simulink model "deadbeat_smm_with_lqr"  (R2015a)
settings: Solver=FixedStepDiscrete  SolverMode=SingleTasking  StartTime=0.0  StopTime=inf  FixedStep=sample_time  RelTol=1e-3
undefined symbols (not defined in the file or in its folder): A_kalman_fourbar_gear, A_kalman_transverse, A_kalman_vertical, A_lpf_accelerometer, A_lpf_fourbar_angles, A_lpf_imu, A_lpf_lateral_angle, B1_lpf_accelerometer, B1_lpf_fourbar_angles, B1_lpf_imu, B1_lpf_lateral_angle, B2_lpf_accelerometer, B2_lpf_fourbar_angles, B2_lpf_imu, B2_lpf_lateral_angle, B_dx_versus_x0, B_kalman_fourbar_gear, B_kalman_transverse, B_kalman_vertical, backwards_K_sag_of_t, backwards_P_sag_of_t, C_kalman_fourbar_gear, C_kalman_transverse, C_kalman_vertical, com_leg_motor, com_torso, contact_threshold, control_start_time, d_ankle_to_foot, d_vertical_com, desired_com_forward_velocity, desired_com_lateral_velocity, desired_initial_leg_roll_left, desired_initial_leg_roll_right, desired_stance_beta2, desired_standing_torso_pitch, desired_standing_torso_roll, desired_standing_z, desired_torso_pitch, desired_torso_roll, Discrete, enable_bouncing, fcut_contact, fdesignblkfcn, forward_dx_of_dxstar, forward_x_of_dxstar, g, gcbh, HIP_MTR_MAX_CONT_TORQUE, HIP_MTR_MAX_TORQUE, i_leg_motor, i_robot, i_torso, initial_dx_estimate, initial_dy_estimate, initial_dz_estimate, initial_leg_selection, initial_z_estimate, k_lateral_accel_for_torso_roll, k_lateral_swing_on_boom ... (+77)
libraries: simulink x21, ctrlSharedLib x7, dsparch4 x3
(part 1 of 5)
settings Model: CovSFcnEnable=off  Creator=wmartin  LastModifiedBy=wmartin
settings SolverCC: EnableConcurrentExecution=on
settings DataIOCC: LimitDataPoints=off  MaxDataPoints=1000000000  SaveFormat=StructureWithTime  SignalLogging=off  DSMLogging=off  VisualizeSimOutput=off
settings OptimizationCC: BlockReduction=off  OptimizeBlockIOStorage=off  BufferReuse=off  GlobalBufferReuse=off  ExpressionFolding=off  ExpressionDepthLimit=2147483647  LocalBlockOutputs=off  SimCompilerOptimization=on
settings DebuggingCC: UnderspecifiedInitializationDetection=Classic  MergeDetectMultiDrivingBlocksExec=none  SolverPrmCheckMsg=warning  StateNameClashWarn=warning
settings HardwareCC: ProdIntDivRoundTo=Zero  ProdEndianess=LittleEndian  ProdLongLongMode=on  ProdHWDeviceType=Generic->32-bit x86 compatible
settings ModelReferenceCC: UpdateModelReferenceTargets=IfOutOfDate  ModelReferenceNumInstancesAllowed=Single  ModelReferenceMinAlgLoopOccurrences=on
settings RTWCC: SystemTargetFile=slrt.tlc  TemplateMakefile=slrt_default_tmf  Description=Simulink Real-Time  RTWVerbose=off  RTWCompilerOptimization=on
settings CodeAppCC: MaxIdLength=256
settings SimulinkRealTimeCC: GeneratePreprocessorConditionals=Disable all  RL32LogBufSizeModifier=1e8

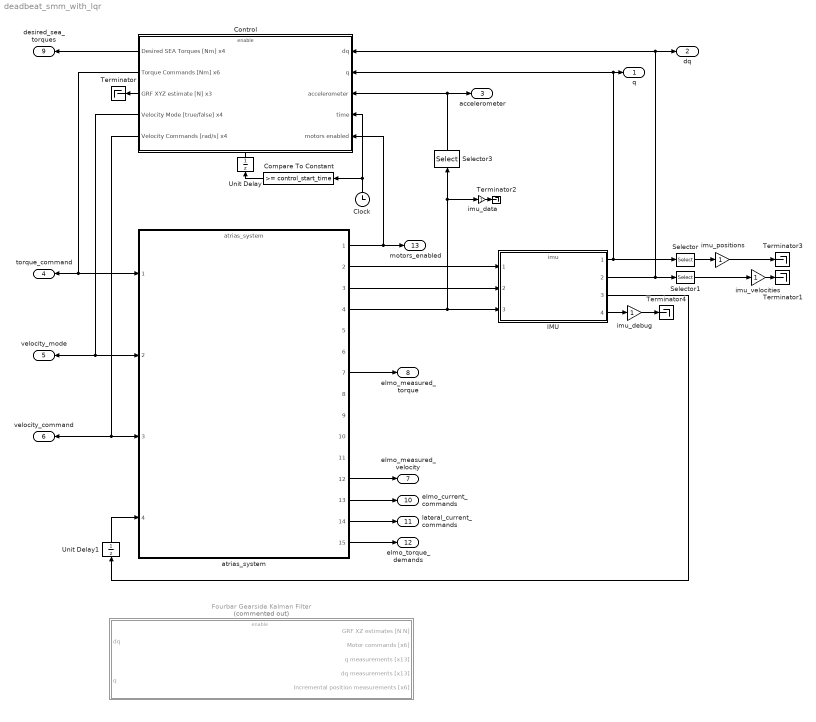
== system deadbeat_smm_with_lqr ==
  Clock : Clock
  Compare To Constant : simulink/Logic and Bit Operations/Compare To Constant  relop=>=  const=control_start_time  OutDataTypeStr=boolean
  Control : Subsystem
  Fourbar Gearside Kalman Filter : Subsystem  Commented=on
  IMU : ModelReference  ModelNameDialog=imu  SimulationMode=Normal  ModelReferenceVersion=1.2455  CopyOfModelName=imu  DefaultDataLogging=on
  Selector : Selector  InputPortWidth=13  Indices=[11 12 13]
  Selector1 : Selector  InputPortWidth=13  Indices=[11 12 13]
  Selector3 : Selector  InputPortWidth=9  Indices=[4 5 6]
  Terminator{,1..4} (5 alike) : Terminator
  Unit Delay : UnitDelay  SampleTime=-1
  Unit Delay1 : UnitDelay  SampleTime=-1
  atrias_system : ModelReference  ModelNameDialog=atrias_system  SimulationMode=Normal  ModelReferenceVersion=1.2965  CopyOfModelName=atrias_system  DefaultDataLogging=on
  imu_data : Gain
  imu_debug : Gain
  imu_positions : Gain
  imu_velocities : Gain
  q : Outport  SampleTime=sample_time
  dq : Outport  Port=2  SampleTime=sample_time
  accelerometer : Outport  Port=3  SampleTime=sample_time
  torque_command : Outport  Port=4  SampleTime=sample_time
  velocity_mode : Outport  Port=5  SampleTime=sample_time
  velocity_command : Outport  Port=6  SampleTime=sample_time
  elmo_measured_velocity : Outport  Port=7  SampleTime=sample_time
  elmo_measured_torque : Outport  Port=8  SampleTime=sample_time
  desired_sea_torques : Outport  Port=9  SampleTime=sample_time
  elmo_current_commands : Outport  Port=10  SampleTime=sample_time
  lateral_current_commands : Outport  Port=11  SampleTime=sample_time
  elmo_torque_demands : Outport  Port=12  SampleTime=sample_time
  motors_enabled : Outport  Port=13  SampleTime=sample_time
  wires:
  Compare To Constant/1 -> Unit Delay/1
  imu_data/1 -> Terminator2/1
  imu_velocities/1 -> Terminator1/1
  imu_positions/1 -> Terminator3/1
  imu_debug/1 -> Terminator4/1
  IMU/4 -> imu_debug/1
  Selector/1 -> imu_positions/1
  Selector1/1 -> imu_velocities/1
  atrias_system/2 -> IMU/1
  IMU/1 -> Selector/1, Control/2(q), q/1
  Control/2(Torque Commands [Nm] x6) -> atrias_system/1, torque_command/1
  atrias_system/3 -> IMU/2
  atrias_system/4 -> Selector3/1, imu_data/1, IMU/3
  IMU/3 -> Unit Delay1/1
  Unit Delay/1 -> Control/Enable
  IMU/2 -> Selector1/1, Control/1(dq), dq/1
  Control/5(Velocity Commands [rad/s] x4) -> velocity_command/1, atrias_system/3
  Control/4(Velocity Mode [true/false] x4) -> velocity_mode/1, atrias_system/2
  Selector3/1 -> Control/3(accelerometer), accelerometer/1
  Control/1(Desired SEA Torques [Nm] x4) -> desired_sea_torques/1
  Clock/1 -> Control/4(time), Compare To Constant/1
  Control/3(GRF XYZ estimate [N] x3) -> Terminator/1
  atrias_system/15 -> elmo_torque_demands/1
  atrias_system/14 -> lateral_current_commands/1
  atrias_system/13 -> elmo_current_commands/1
  atrias_system/12 -> elmo_measured_velocity/1
  atrias_system/7 -> elmo_measured_torque/1
  atrias_system/1 -> Control/5(motors enabled), motors_enabled/1
  Unit Delay1/1 -> atrias_system/4

== system deadbeat_smm_with_lqr/Control ==
  dq : Inport
  q : Inport  Port=2
  accelerometer : Inport  Port=3
  time : Inport  Port=4
  motors enabled : Inport  Port=5
  Enable : EnablePort  StatesWhenEnabling=reset  PropagateVarSize=During execution  ShowOutputPort=on
  Actuator Control : ModelReference  ModelNameDialog=actuator_control  SimulationMode=Normal  ModelReferenceVersion=1.1251  CopyOfModelName=actuator_control  DefaultDataLogging=on
  Behavior Control : Subsystem
  Compute Body Frame Accelerations : Subsystem
  Detect Change : simulink/Logic and Bit Operations/Detect Change  vinit=0  InputProcessing=Inherited  OutDataTypeStr=boolean
  Filter Velocities : Subsystem
  Mux : Mux
  Desired SEA Torques [Nm] x4 : Outport  InitialOutput=[0 0 0 0]
  Torque Commands [Nm] x6 : Outport  Port=2  InitialOutput=[0 0 0 0 0 0]
  GRF XYZ estimate [N] x3 : Outport  Port=3  InitialOutput=[0 0 0]
  Velocity Mode [true/false] x4 : Outport  Port=4  InitialOutput=[false false false false]
  Velocity Commands [rad/s] x4 : Outport  Port=5  InitialOutput=[0 0 0 0]
  wires:
  Behavior Control/1(Torque Commands [Nm] x6) -> Actuator Control/2
  Behavior Control/2(Velocity Commands [rad/s] x4) -> Actuator Control/3
  Behavior Control/3(Stance / Swing Control [1/0] x4) -> Actuator Control/4
  time/1 -> Actuator Control/5, Behavior Control/5(time)
  Detect Change/1 -> Mux/1, Mux/2, Mux/3, Mux/4
  motors enabled/1 -> Detect Change/1
  Mux/1 -> Actuator Control/1
  Actuator Control/4 -> Desired SEA Torques [Nm] x4/1
  Enable/1 -> Behavior Control/1(Enabled [true/false])
  Compute Body Frame Accelerations/1(accelerations [m/s^2] x3) -> Behavior Control/2(Body XYZ Acceleration [m/s^2] x3)
  accelerometer/1 -> Compute Body Frame Accelerations/1(accelerometer [g] x3)
  Actuator Control/3 -> Velocity Commands [rad/s] x4/1
  Actuator Control/2 -> Velocity Mode [true/false] x4/1
  dq/1 -> Actuator Control/7, Filter Velocities/1(raw dq)
  Filter Velocities/1(filtered dq) -> Behavior Control/3(dq)
  Behavior Control/4(GRF XYZ estimates [N N N]) -> GRF XYZ estimate [N] x3/1
  Actuator Control/1 -> Torque Commands [Nm] x6/1
  q/1 -> Actuator Control/6, Behavior Control/4(q)

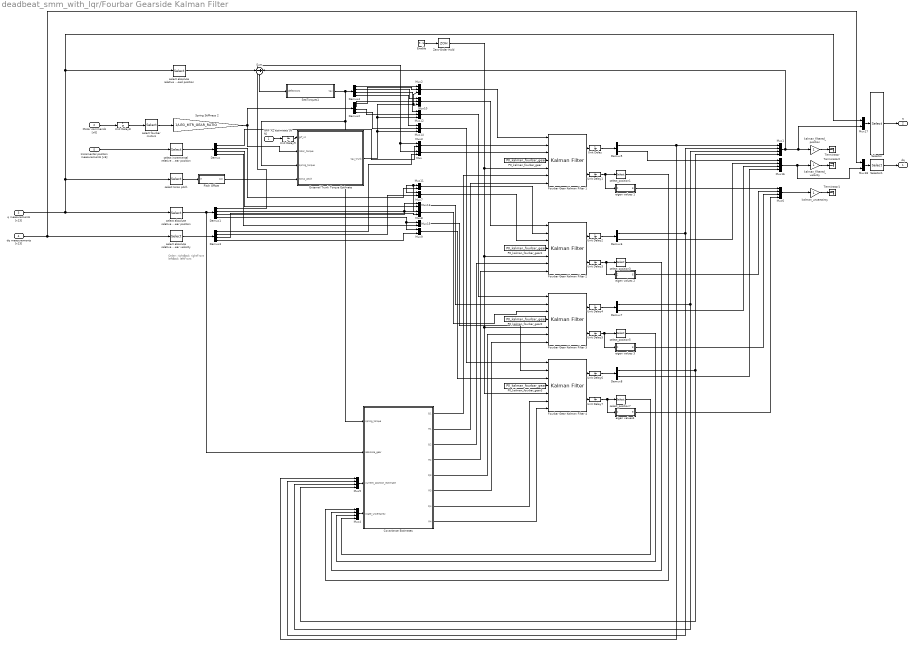
== system deadbeat_smm_with_lqr/Fourbar Gearside Kalman Filter ==
  note: Order:
      | rightBack
      | rightFront
      | leftBack
      | leftFront
  GRF XZ estimates [N N] : Inport  SampleTime=sample_time
  Motor commands [x6] : Inport  Port=2  SampleTime=sample_time
  q measurements [x13] : Inport  Port=3  SampleTime=sample_time
  dq measurements [x13] : Inport  Port=4  SampleTime=sample_time
  Incremental position measurements [x6] : Inport  Port=5  SampleTime=sample_time
  Enable : EnablePort  ShowOutputPort=on
  Covariance Estimates : MATLAB Function  TreatAsAtomicUnit=on
  Demux{,1..4} (5 alike) : Demux
  Demux{5..8} (4 alike) : Demux  Outputs=2
  External Trunk Torque Estimate : MATLAB Function  TreatAsAtomicUnit=on
  Fourbar Gear Kalman Filter {1..4} (4 alike) : ctrlSharedLib/Kalman Filter  TimeDomain=Discrete-Time  UseCurrentEstimator=on  ModelSource=Individual A, B, C, D matrices  ModelSourceVariable=A_kf  A=A_kalman_fourbar_gear  B=B_kalman_fourbar_gear  C=C_kalman_fourbar_gear  D=0  NumberOfStates=2  NumberOfInputs=1  NumberOfOutputs=2  InitialEstimateSource=Input port  X0=initial_dx_estimate  P0=P0_kalman_transverse  UseK=off  UseGH=on  NumberOfProcessNoiseInputs=1  G=G_kalman_fourbar_gear  TimeInvariantG=on  H=0  TimeInvariantH=on  Q=1  TimeInvariantQ=off  R=1  TimeInvariantR=off  N=0  TimeInvariantN=on  AddInputPort=on  AddEnablePort=off  ExternalReset=Either  OutputEstimatedY=off  OutputP=on  Ts=sample_time
  Mux{,3,7..9,11,13,15,17..18} (10 alike) : Mux  Inputs=2
  Mux{1,4..6,16} (5 alike) : Mux
  Mux{2,10,12,14} (4 alike) : Mux  Inputs=3
  P0_kalman_fourbar_gear{,1..3} (4 alike) : Constant  Value=P0_kalman_fourbar_gear
  Pitch Offset : Subsystem
  SeaTorques1 : MATLAB Function  TreatAsAtomicUnit=on
  Selector : Selector  InputPortWidth=17  Indices=[1 14 3 15 5 16 7 17 9 10 11 12 13]
  Selector1 : Selector  InputPortWidth=17  Indices=[1 14 3 15 5 16 7 17 9 10 11 12 13]
  Spring Stiffness 2 : Gain  Gain=1/LEG_MTR_GEAR_RATIO
  Sum : Sum  Inputs=-|+
  Terminator : Terminator
  Terminator1 : Terminator
  Terminator2 : Terminator
  Unit Delay{,1..9} (10 alike) : UnitDelay  SampleTime=-1
  Zero-Order Hold : ZeroOrderHold  SampleTime=sample_time
  eigen values 1 : MATLAB Function  TreatAsAtomicUnit=on
  eigen values 2 : MATLAB Function  TreatAsAtomicUnit=on
  eigen values 3 : MATLAB Function  TreatAsAtomicUnit=on
  "eigen values4 " : MATLAB Function  TreatAsAtomicUnit=on
  kalman_filtered_position : Gain
  kalman_filtered_velocity : Gain
  kalman_uncertainty : Gain
  select absolute relative gear position : Selector  InputPortWidth=13  Indices=[2 4 6 8]
  select absolute relative gear velocity : Selector  InputPortWidth=13  Indices=[2 4 6 8]
  select absolute relative load position : Selector  InputPortWidth=13  Indices=[2 4 6 8]
  select fourbar motors : Selector  InputPortWidth=6  Indices=[1 2 3 4]
  select incremental relative gear position : Selector  InputPortWidth=6  Indices=[1 2 3 4]
  select torso pitch : Selector  InputPortWidth=13  Indices=[13]
  select_position{1,3,5,7} (4 alike) : Selector  NumberOfDimensions=2  InputPortWidth=2  IndexOptions=Index vector (dialog),Index vector (dialog)  Indices=[1],[1]  OutputSizes=1,1
  dq : Outport
  q : Outport  Port=2
  wires:
  select incremental relative gear position/1 -> Demux/1
  q measurements [x13]/1 -> select absolute relative gear position/1, Mux17/1, select absolute relative load position/1, select torso pitch/1
  Incremental position measurements [x6]/1 -> select incremental relative gear position/1
  Motor commands [x6]/1 -> Unit Delay8/1
  select fourbar motors/1 -> Spring Stiffness 2/1
  P0_kalman_fourbar_gear/1 -> Fourbar Gear Kalman Filter 1/4
  Mux/1 -> Fourbar Gear Kalman Filter 1/3
  select absolute relative gear velocity/1 -> Demux3/1
  dq measurements [x13]/1 -> Mux18/1, select absolute relative gear velocity/1
  Demux3/1 -> Mux/2
  GRF XZ estimates [N N]/1 -> Unit Delay9/1
  SeaTorques1/1(tau) -> Demux4/1, External Trunk Torque Estimate/3(spring_torque), Covariance Estimates/1(spring_torque)
  Fourbar Gear Kalman Filter 1/1 -> Unit Delay/1
  Demux5/1 -> Mux1/1, Mux5/1
  Mux1/1 -> Sum/2, Mux17/2, kalman_filtered_position/1
  select absolute relative load position/1 -> Sum/1
  Sum/1 -> SeaTorques1/1(deflections)
  External Trunk Torque Estimate/1(tau_trunk) -> Mux2/3, Mux10/3, Mux12/3, Mux14/3
  Demux4/1 -> Mux2/1
  Demux2/1 -> Mux2/2
  Mux2/1 -> Fourbar Gear Kalman Filter 1/1
  Demux/1 -> Mux3/2
  Demux1/1 -> Mux3/1, Mux/1
  Mux3/1 -> Fourbar Gear Kalman Filter 1/2
  Fourbar Gear Kalman Filter 1/2 -> Unit Delay1/1
  Mux4/1 -> Covariance Estimates/4(state_uncertainty)
  select absolute relative gear position/1 -> Covariance Estimates/2(absolute_gear), Demux1/1
  Mux5/1 -> Covariance Estimates/3(current_position_estimate)
  Covariance Estimates/1(Q1) -> Fourbar Gear Kalman Filter 1/6
  Covariance Estimates/2(R1) -> Fourbar Gear Kalman Filter 1/7
  select torso pitch/1 -> Pitch Offset/1(in)
  select_position1/1 -> Mux4/1
  P0_kalman_fourbar_gear1/1 -> Fourbar Gear Kalman Filter 2/4
  Fourbar Gear Kalman Filter 2/1 -> Unit Delay2/1
  Fourbar Gear Kalman Filter 2/2 -> Unit Delay3/1
  P0_kalman_fourbar_gear2/1 -> Fourbar Gear Kalman Filter 3/4
  Fourbar Gear Kalman Filter 3/1 -> Unit Delay4/1
  Fourbar Gear Kalman Filter 3/2 -> Unit Delay5/1
  P0_kalman_fourbar_gear3/1 -> Fourbar Gear Kalman Filter 4/4
  Fourbar Gear Kalman Filter 4/1 -> Unit Delay6/1
  Fourbar Gear Kalman Filter 4/2 -> Unit Delay7/1
  Covariance Estimates/3(Q2) -> Fourbar Gear Kalman Filter 2/6
  Covariance Estimates/5(Q3) -> Fourbar Gear Kalman Filter 3/6
  Covariance Estimates/7(Q4) -> Fourbar Gear Kalman Filter 4/6
  Covariance Estimates/4(R2) -> Fourbar Gear Kalman Filter 2/7
  Covariance Estimates/6(R3) -> Fourbar Gear Kalman Filter 3/7
  Covariance Estimates/8(R4) -> Fourbar Gear Kalman Filter 4/7
  select_position3/1 -> Mux4/2
  select_position5/1 -> Mux4/3
  select_position7/1 -> Mux4/4
  Demux6/1 -> Mux5/2, Mux1/2
  Demux7/1 -> Mux1/3, Mux5/3
  Demux8/1 -> Mux1/4, Mux5/4
  kalman_filtered_position/1 -> Terminator/1
  Enable/1 -> Zero-Order Hold/1
  Mux7/1 -> Fourbar Gear Kalman Filter 2/3
  Mux8/1 -> Fourbar Gear Kalman Filter 3/3
  Mux9/1 -> Fourbar Gear Kalman Filter 4/3
  Mux10/1 -> Fourbar Gear Kalman Filter 2/1
  Mux11/1 -> Fourbar Gear Kalman Filter 2/2
  Mux13/1 -> Fourbar Gear Kalman Filter 3/2
  Mux12/1 -> Fourbar Gear Kalman Filter 3/1
  Mux15/1 -> Fourbar Gear Kalman Filter 4/2
  Mux14/1 -> Fourbar Gear Kalman Filter 4/1
  Demux3/2 -> Mux7/2
  Demux3/3 -> Mux8/2
  Demux3/4 -> Mux9/2
  Demux1/2 -> Mux7/1, Mux11/1
  Demux1/3 -> Mux13/1, Mux8/1
  Demux1/4 -> Mux9/1, Mux15/1
  Demux/2 -> Mux11/2
  Demux/3 -> Mux13/2
  Demux/4 -> Mux15/2
  Demux4/2 -> Mux10/1
  Demux4/3 -> Mux12/1
  Demux4/4 -> Mux14/1
  Demux2/2 -> Mux10/2
  Demux2/3 -> Mux12/2
  Demux2/4 -> Mux14/2
  kalman_uncertainty/1 -> Terminator1/1
  Mux6/1 -> kalman_uncertainty/1
  kalman_filtered_velocity/1 -> Terminator2/1
  Mux16/1 -> Mux18/2, kalman_filtered_velocity/1
  Demux5/2 -> Mux16/1
  Demux6/2 -> Mux16/2
  Demux7/2 -> Mux16/3
  Demux8/2 -> Mux16/4
  Zero-Order Hold/1 -> Fourbar Gear Kalman Filter 4/5, Fourbar Gear Kalman Filter 3/5, Fourbar Gear Kalman Filter 2/5, Fourbar Gear Kalman Filter 1/5
  Unit Delay1/1 -> eigen values 1/1(Z), select_position1/1
  Unit Delay3/1 -> eigen values 2/1(Z), select_position3/1
  Unit Delay4/1 -> Demux7/1
  Unit Delay7/1 -> "eigen values4 "/1(Z), select_position7/1
  Unit Delay6/1 -> Demux8/1
  Spring Stiffness 2/1 -> Demux2/1, External Trunk Torque Estimate/2(rotor_torque)
  Unit Delay5/1 -> eigen values 3/1(Z), select_position5/1
  eigen values 1/1(E) -> Mux6/1
  eigen values 2/1(E) -> Mux6/2
  eigen values 3/1(E) -> Mux6/3
  "eigen values4 "/1(E) -> Mux6/4
  Unit Delay/1 -> Demux5/1
  Unit Delay2/1 -> Demux6/1
  Mux17/1 -> Selector/1
  Selector/1 -> q/1
  Selector1/1 -> dq/1
  Mux18/1 -> Selector1/1
  Unit Delay8/1 -> select fourbar motors/1
  Unit Delay9/1 -> External Trunk Torque Estimate/1(grf_xz)
  Pitch Offset/1(out) -> External Trunk Torque Estimate/4(torso_pitch)

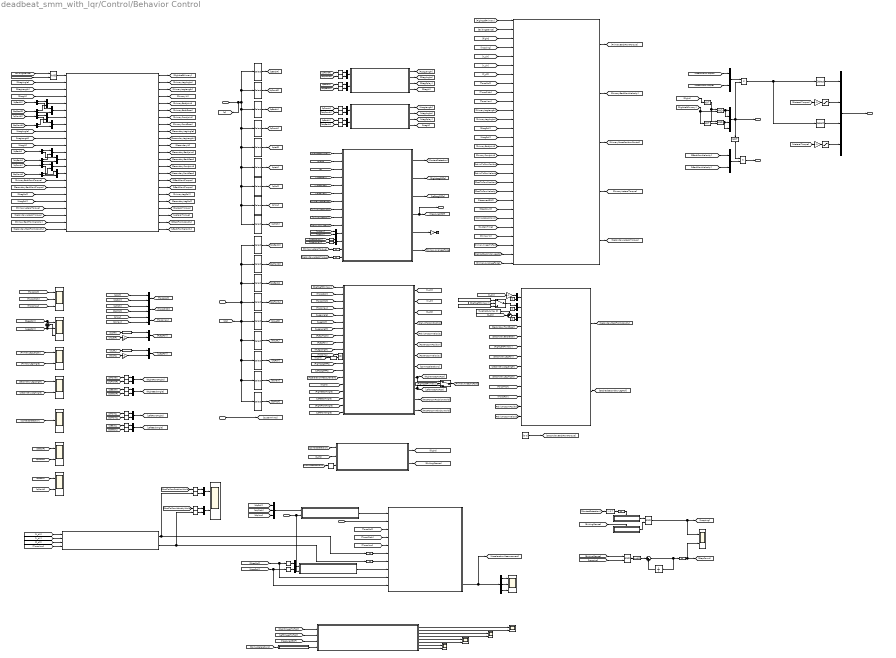
== system deadbeat_smm_with_lqr/Control/Behavior Control ==
  note: Knee Torque Estimation
  note: Acceleration Measurement
  note: Logging
  note: Contact Estimation
  note: Angle Conversions
  note: Motor Order:
      |
      | backR
      | frontR
      | latR
      | backL
      | frontL
      | latL
  note: q Order:
      |
      | backJointR
      | backGearR
      | frontJointR
      | frontGearR
      |
      | backJointL
      | backGearL
      | frontJointL
      | frontGearL
      |
      | latR
      | latL
      |
      | torsoRoll
      | torsoYaw
      | torsoPitch
  note: Inputs
  note: Primary Leg + Lateral Behavior
  note: Secondary Leg Behavior
  note: Torque Commands
  note: Leg/Spring Measurements
  note: Force Estimation
  note: Position & Velocity Estimation
  note: Begin Control
  note: Signal Routing
  Enabled [true/false] : Inport
  Body XYZ Acceleration [m/s^2] x3 : Inport  Port=2
  dq : Inport  Port=3
  q : Inport  Port=4
  time : Inport  Port=5
  At Least One Stance Detected : Subsystem
  Atrias Swing control : Subsystem
  COM Acceleration Measurement : Scope  NumInputPorts=3
      settings: YMin=-10~-12.5~-15  YMax=7.5~7.5~15  SaveName=ScopeData34  SampleInput=on
  COM World Frame X : Scope  NumInputPorts=2
      settings: TimeRange=3.175000000000004  YMin=-0.004~-0.175  YMax=0.02~0.225  SaveName=ScopeData35  SampleInput=on
  Compare To Constant : simulink/Logic and Bit Operations/Compare To Constant  relop=>  const=0.7  OutDataTypeStr=boolean
  Compute COM Translational Acceleration (IMU uses non-rotating measurement frame) : MATLAB Function  TreatAsAtomicUnit=on
  Compute Forces1 : Subsystem
  Compute World Frame COM Coordinates from Yawed Frame : MATLAB Function  TreatAsAtomicUnit=on
  Constant : Constant  Value=[0 0]
  Constant1 : Constant  Value=[lateral_target_position_right, 0]
  Constant2 : Constant  Value=[lateral_target_position_left, 0]
  Constant3 : Constant  Value=[z_retract_swing, 0]
  Constant4 : Constant  Value=0
  Constant5 : Constant  Value=0
  Constant6 : Constant  Value=0
  Contact : Scope
      settings: YMin=0.3  YMax=0.9  SaveName=ScopeData11  SampleInput=on
  Contact State Machine : Subsystem
  Data Type Conversion : DataTypeConversion  OutDataTypeStr=uint32
  Demux : Demux  Outputs=3
  Demux{3..10} (8 alike) : Demux  Outputs=2
  Estimate Angular Accelerations2 : Subsystem
  Estimate Angular Accelerations3 : Subsystem
  Exited Stance : Subsystem
  Force Estimation : Subsystem
  Gain{,1..2,12..13} (5 alike) : Gain  Gain=-1
  Hopping / Steps : Scope  NumInputPorts=2
      settings: YMin=1~1  YMax=1~1  SaveName=ScopeData33  SampleInput=on
  Knee Torques : MATLAB Function  TreatAsAtomicUnit=on
  L Knee Torques from Accelerometer : Scope  NumInputPorts=2
      settings: YMin=-1000~-1250  YMax=1500~2000  SaveName=ScopeData42  SampleInput=on
  L Knee Torques from Forward Dynamics : Scope  NumInputPorts=2
      settings: YMin=-75~-220  YMax=250~0  SaveName=ScopeData43  SampleInput=on
  L Leg Calculator : Subsystem
  Left Lateral Torque Saturation : Saturate  UpperLimit=max_torque_lateral  LowerLimit=-max_torque_lateral
      settings: AttributesFormatString=Top: %<UpperLimit>\nBottom: %<LowerLimit>
  Left Leg Fourbar Positions : Scope  NumInputPorts=2
      settings: YMin=4.05~2.275  YMax=4.17~2.375  SaveName=ScopeData17  SampleInput=on
  Logical Operator : Logic  IconShape=distinctive  AllPortsSameDT=off  OutDataTypeStr=boolean
  Logical Operator{1,3,5,7} (4 alike) : Logic  AllPortsSameDT=off  OutDataTypeStr=boolean
  Logical Operator2 : Logic  Operator=OR  AllPortsSameDT=off  OutDataTypeStr=boolean
  Logical Operator{4,6,8..9} (4 alike) : Logic  Operator=NOT  AllPortsSameDT=off  OutDataTypeStr=boolean
  Mux : Mux
  Mux{1..2,4..27,29..33} (31 alike) : Mux  Inputs=2
  Mux28 : Mux  Inputs=3
  Mux3 : Mux
  Primary Leg Length / Angle : Scope  NumInputPorts=2
      settings: YMin=0.3~0  YMax=0.9~3.5  SaveName=ScopeData21  SampleInput=on
  Primary Secondary Leg Swap : Subsystem
  Primary and Lateral Behavior : Subsystem
  Product : Product
  Product1 : Product
  R Knee Torques from Accelerometer : Scope  NumInputPorts=2
      settings: YMin=0.95~0.95  YMax=1.05~1.05  SaveName=ScopeData41  SampleInput=on
  R Knee Torques from Forward Dynamics : Scope  NumInputPorts=2
      settings: YMin=0.95~0.95  YMax=1.05~1.05  SaveName=ScopeData40  SampleInput=on
  R Leg Calculator : Subsystem
  Right Lateral Torque Saturation : Saturate  UpperLimit=max_torque_lateral  LowerLimit=-max_torque_lateral
      settings: AttributesFormatString=Top: %<UpperLimit>\nBottom: %<LowerLimit>
  Right Left Symmetry Leg Roll : Scope  NumInputPorts=3
      settings: YMin=-0.2~-0.5~-0.5  YMax=1.3~1.8~0.5  SaveName=ScopeData19  SampleInput=on
  Right Leg Fourbar Positions : Scope  NumInputPorts=2
      settings: YMin=3.19015~1.00606  YMax=3.99645~2.79375  SaveName=ScopeData16
  Roll Pitch Yaw : Scope  NumInputPorts=3
      settings: YMin=-1000~-5~-5  YMax=1000~5~5  SampleInput=on
  Secondary Leg Length / Angle : Scope  NumInputPorts=2
      settings: YMin=-1~-0.8  YMax=1~1.4  SaveName=ScopeData22  SampleInput=on
  Selector : Selector  InputPortWidth=4  Indices=[1 2]
  Selector1 : Selector  InputPortWidth=13  Indices=[10]
  Selector10 : Selector  InputPortWidth=13  Indices=[7 8]
  Selector11 : Selector  InputPortWidth=13  Indices=[9]
  Selector12 : Selector  InputPortWidth=13  Indices=[1 2]
  Selector13 : Selector  InputPortWidth=13  Indices=[3 4]
  Selector{14..17,19,24..27,29..37} (18 alike) : Selector  InputPortWidth=2  Indices=[1]
  Selector18 : Selector  InputPortWidth=13  Indices=[13]
  Selector2 : Selector  InputPortWidth=13  Indices=[5 6]
  Selector20 : Selector  InputPortWidth=13  Indices=[13]
  Selector21 : Selector  InputPortWidth=13  Indices=[11]
  Selector22 : Selector  InputPortWidth=13  Indices=[12]
  Selector23 : Selector  InputPortWidth=13  Indices=[11]
  Selector28 : Selector  InputPortWidth=13  Indices=[12]
  Selector3 : Selector  InputPortWidth=4  Indices=[3 4]
  Selector38 : Selector  InputPortWidth=3  Indices=[3]
  Selector4 : Selector  InputPortWidth=13  Indices=[7 8]
  Selector41 : Selector  InputPortWidth=2  Indices=[2]
  Selector42 : Selector  InputPortWidth=2  Indices=[2]
  Selector{43..46} (4 alike) : Selector  InputPortWidth=3  Indices=[1]
  Selector5 : Selector  InputPortWidth=13  Indices=[9]
  Selector6 : Selector  InputPortWidth=13  Indices=[1 2]
  Selector7 : Selector  InputPortWidth=13  Indices=[3 4]
  Selector8 : Selector  InputPortWidth=13  Indices=[10]
  Selector9 : Selector  InputPortWidth=13  Indices=[5 6]
  State Estimation : Subsystem
  Sum1 : Sum  Inputs=|++  OutMin=0
  Sum2 : Sum  Inputs=-+|
  Sum3 : Sum  Inputs=-|+
  Switch : Switch  Criteria=u2 ~= 0
  Switch1 : Switch  Criteria=u2 ~= 0
  Terminator6 : Terminator
  Unit Delay : UnitDelay  SampleTime=-1
  Unit Delay{1..6} (6 alike) : UnitDelay  SampleTime=sample_time
  lateral_coordinates : Fcn  Expr=pi/2-u
  lateral_coordinates1 : Fcn  Expr=pi/2-u
  torso_roll_acceleration : Gain
  Torque Commands [Nm] x6 : Outport  OutputWhenDisabled=reset  InitialOutput=[0 0 0 0 0 0]
  Velocity Commands [rad/s] x4 : Outport  Port=2  OutputWhenDisabled=reset  InitialOutput=[0 0 0 0 0 0]
  Stance / Swing Control [1/0] x4 : Outport  Port=3  OutputWhenDisabled=reset  InitialOutput=[0 0 0 0 0 0]
  GRF XYZ estimates [N N N] : Outport  Port=4  OutputWhenDisabled=reset  InitialOutput=[0 0 0 0 0 0]
  wires:
  [PrimaryKneesToFoot] -> Primary and Lateral Behavior/26(Primary Knees to Foot [m] x6)
  Selector38/1 -> Contact State Machine/3(ddZ [m/s^2])
  [ComAccelerations] -> Selector38/1
  Mux26/1 -> [LeftBackAngle]
  Mux27/1 -> [LeftFrontAngle]
  Mux17/1 -> [RightBackAngle]
  Mux18/1 -> [RightFrontAngle]
  Selector36/1 -> Mux26/1
  Selector37/1 -> Mux26/2
  Selector35/1 -> Mux27/2
  Selector34/1 -> Mux27/1
  [dqFrontL] -> Selector35/1
  [qFrontL] -> Selector34/1
  [dqBackL] -> Selector37/1
  [qBackL] -> Selector36/1
  Selector32/1 -> Mux17/1
  Selector33/1 -> Mux17/2
  Selector31/1 -> Mux18/2
  Selector30/1 -> Mux18/1
  [dqFrontR] -> Selector31/1
  [qFrontR] -> Selector30/1
  [dqBackR] -> Selector33/1
  [qBackR] -> Selector32/1
  Knee Torques/7(left_front_knee_torques_from_accelerometer) -> L Knee Torques from Accelerometer/1
  Knee Torques/8(left_back_knee_torques_from_accelerometer) -> L Knee Torques from Accelerometer/2
  Knee Torques/6(left_back_knee_torques_from_fd) -> L Knee Torques from Forward Dynamics/2
  Knee Torques/5(left_front_knee_torques_from_fd) -> L Knee Torques from Forward Dynamics/1
  Knee Torques/4(right_back_knee_torques_from_accelerometer) -> R Knee Torques from Accelerometer/2
  Knee Torques/3(right_front_knee_torques_from_accelerometer) -> R Knee Torques from Accelerometer/1
  Knee Torques/2(right_back_knee_torques_from_fd) -> R Knee Torques from Forward Dynamics/2
  Knee Torques/1(right_front_knee_torques_from_fd) -> R Knee Torques from Forward Dynamics/1
  Compute Forces1/1(XYZ Force) -> Knee Torques/4(grf_from_accelerometer)
  [MeasuredGRF] -> Knee Torques/3(grf_from_seas)
  [LeftKneesToFoot] -> Knee Torques/2(left_knees_to_foot)
  [RightKneesToFoot] -> Knee Torques/1(right_knees_to_foot)
  [ComAccelerations] -> Compute Forces1/1(XYZ Acceleration)
  Constant/1 -> [SecondaryBackFrontTorque]
  Product1/1 -> Selector/1, Selector3/1
  Mux8/1 -> Product1/1
  [LBackFrontTorque] -> Mux8/2
  [RBackFrontTorque] -> Mux8/1
  Logical Operator9/1 -> Product/1
  Product/1 -> Velocity Commands [rad/s] x4/1
  Primary and Lateral Behavior/2(Primary Back/Front Gear Velocities [rad/s] x2) -> [PrimaryBackFrontVelocity]
  Primary Secondary Leg Swap/23(Left Front/Back Velocity [rad/s rad/s]) -> [LBackFrontVelocity]
  Primary Secondary Leg Swap/22(Right Front/Back Velocity [rad/s rad/s]) -> [RBackFrontVelocity]
  [SecondaryBackFrontVelocity] -> Primary Secondary Leg Swap/23(Secondary Front/Back Velocity [rad/s rad/s])
  [PrimaryBackFrontVelocity] -> Primary Secondary Leg Swap/22(Primary Front/Back Velocity [rad/s rad/s])
  [LBackFrontVelocity] -> Mux6/2
  [RBackFrontVelocity] -> Mux6/1
  Mux6/1 -> Product/2
  Unit Delay1/1 -> At Least One Stance Detected/Enable
  Exited Stance/1(Takeoff?) -> Logical Operator3/2
  At Least One Stance Detected/1(Stance?) -> Logical Operator3/1
  Compare To Constant/1 -> Unit Delay1/1
  [ContactDetection] -> Compare To Constant/1
  Mux3/1 -> Stance / Swing Control [1/0] x4/1, Product1/2, Logical Operator9/1
  Mux/1 -> Torque Commands [Nm] x6/1
  Selector3/1 -> Mux/3
  Selector/1 -> Mux/1
  [PrimaryW] -> Primary and Lateral Behavior/25(Primary Leg Width [m])
  [RightLeftPrimary] -> Logical Operator5/2, Logical Operator8/1
  Logical Operator8/1 -> Logical Operator7/2
  Logical Operator7/1 -> Mux3/3, Mux3/4
  Logical Operator6/1 -> Logical Operator5/1, Logical Operator7/1
  Logical Operator5/1 -> Mux3/1, Mux3/2
  [flight] -> Logical Operator6/1
  [SystemTime] -> Primary and Lateral Behavior/24(System Time [s])
  time/1 -> [SystemTime]
  [ComAccelerations] -> Primary and Lateral Behavior/23(COM XYZ Acceleration [m/s^2] x3)
  [qFrontL] -> Left Leg Fourbar Positions/2
  [qBackL] -> Left Leg Fourbar Positions/1
  [qFrontR] -> Right Leg Fourbar Positions/2
  [qBackR] -> Right Leg Fourbar Positions/1
  [dqYaw] -> Mux21/2
  [qYaw] -> Mux21/1
  [qPitch] -> Mux7/1
  [qRoll] -> Mux23/1
  dq/1 -> Selector9/1, Selector13/1, Selector12/1, Selector8/1, Selector22/1, Selector20/1, Selector21/1, Selector11/1, [dq], Selector10/1
  Selector21/1 -> [dqRoll]
  Selector22/1 -> [dqYaw]
  Selector20/1 -> [dqPitch]
  Selector10/1 -> [dqFrontL]
  Selector9/1 -> [dqBackL]
  Selector13/1 -> [dqFrontR]
  Selector12/1 -> [dqBackR]
  Selector11/1 -> [dqLatR]
  Selector8/1 -> [dqLatL]
  Gain12/1 -> Mux22/2
  Gain13/1 -> Mux24/2
  lateral_coordinates1/1 -> Mux24/1
  lateral_coordinates/1 -> Mux22/1
  Mux24/1 -> [LLegRoll]
  Mux22/1 -> [RLegRoll]
  [dqLatL] -> Gain13/1
  [qLatL] -> lateral_coordinates1/1
  [dqLatR] -> Gain12/1
  [qLatR] -> lateral_coordinates/1
  [dqPitch] -> Mux7/2
  [dqRoll] -> Mux23/2
  Mux7/1 -> [TorsoPitch]
  Mux23/1 -> [TorsoRoll]
  Mux21/1 -> [TorsoYaw]
  [ContactDetection] -> Contact/1
  [SecondaryLegAngle] -> Secondary Leg Length / Angle/2
  [SecondaryLegLength] -> Secondary Leg Length / Angle/1
  [PrimaryLegAngle] -> Primary Leg Length / Angle/2
  [PrimaryLegLength] -> Primary Leg Length / Angle/1
  Sum3/1 -> Right Left Symmetry Leg Roll/3
  [RLegRoll] -> Right Left Symmetry Leg Roll/1, Sum3/1
  [LLegRoll] -> Right Left Symmetry Leg Roll/2, Sum3/2
  [TorsoRoll] -> Roll Pitch Yaw/1
  [TorsoPitch] -> Roll Pitch Yaw/2
  [TorsoYaw] -> Roll Pitch Yaw/3
  [ExitingStance] -> Primary and Lateral Behavior/2(Exiting Stance [1/0])
  [Z_dZ] -> Contact State Machine/2("[Z dZ] [m m/s]")
  [ContactDetection] -> Contact State Machine/1(Contact Factor [body weight])
  [flight] -> Primary and Lateral Behavior/3(Flight [1/0])
  Contact State Machine/2(Exiting Stance [1/0]) -> [ExitingStance]
  [FootToComPosition] -> Primary and Lateral Behavior/19(Foot to COM Position [m m m])
  [FootToComVelocity] -> Primary and Lateral Behavior/20(Foot to COM Velocity [m m m])
  Contact State Machine/1(flight [1/0]) -> [flight]
  [PrimaryLegAngle] -> Primary and Lateral Behavior/12(Leg Angle [rad rad/s])
  [PrimaryBackJoint] -> Primary and Lateral Behavior/15(Primary Back Load [rad rad/s])
  [RightLeftPrimary] -> Primary and Lateral Behavior/1(Right/Left [1/0])
  [hopping] -> Primary and Lateral Behavior/4(Hopping [1/0])
  [PrimaryLegLength] -> Primary and Lateral Behavior/11(Leg Length [m m/s])
  [PrimaryFrontJoint] -> Primary and Lateral Behavior/16(Primary Front Load [rad rad/s])
  [TorsoPitch] -> Primary and Lateral Behavior/9(Torso Pitch [rad rad/s])
  [PelvisToComPosition] -> Primary and Lateral Behavior/17(Pelvis to COM Position [m m m])
  [PelvisToComVelocity] -> Primary and Lateral Behavior/18(Pelvis to COM Velocity [m m m])
  [X_dX] -> Primary and Lateral Behavior/5("[x, dx] [m, m/s]")
  [Z_dZ] -> Primary and Lateral Behavior/7("[z, dz] [m, m/s]")
  [TorsoRoll] -> Primary and Lateral Behavior/8(Torso Roll [rad rad/s])
  [MeasuredGRF] -> Primary and Lateral Behavior/21(Measured GRF [N N N])
  [StepCount] -> Primary and Lateral Behavior/22(Steps Taken)
  [Y_dY] -> Primary and Lateral Behavior/6("[y,  dy] [m, m/s]")
  [RLegRoll] -> Primary and Lateral Behavior/13(Right Leg Roll [rad rad/s])
  [LLegRoll] -> Primary and Lateral Behavior/14(Left Leg Roll [rad rad/s])
  [TorsoYaw] -> Primary and Lateral Behavior/10(Torso Yaw [rad rad/s])
  Gain1/1 -> Left Lateral Torque Saturation/1
  Gain2/1 -> Right Lateral Torque Saturation/1
  Logical Operator3/1 -> [hopping], Hopping / Steps/1
  Unit Delay4/1 -> Force Estimation/14(Secondary Lateral Torque [Nm])
  Unit Delay3/1 -> Force Estimation/13(Primary Lateral Torque [Nm])
  Selector29/1 -> Mux20/2
  [LLegLength] -> Selector29/1
  Selector19/1 -> Mux20/1
  Primary and Lateral Behavior/4(Primary Lateral Torque [Nm]) -> [PrimaryLateralTorque]
  Primary and Lateral Behavior/5(Secondary Lateral Torque [Nm]) -> [SecondaryLateralTorque]
  Left Lateral Torque Saturation/1 -> Mux/4
  Right Lateral Torque Saturation/1 -> Mux/2
  Primary Secondary Leg Swap/21(Left Lateral Torque [Nm]) -> [LLateralTorque]
  Primary Secondary Leg Swap/20(Right Lateral Torque [Nm]) -> [RLateralTorque]
  [SecondaryLateralTorque] -> Primary Secondary Leg Swap/21(Secondary Lateral Torque [Nm])
  [PrimaryLateralTorque] -> Primary Secondary Leg Swap/20(Primary Lateral Torque [Nm])
  Force Estimation/5(Torso Roll Acceleration [rad/s^2]) -> torso_roll_acceleration/1
  torso_roll_acceleration/1 -> Terminator6/1
  [SecondaryLateralTorque] -> Unit Delay4/1
  [PrimaryLateralTorque] -> Unit Delay3/1
  [SecondaryLegRoll] -> Force Estimation/10(Secondary Leg Roll [rad rad/s])
  Mux20/1 -> Force Estimation/12(Leg Length Right/Left [m m])
  [RLegLength] -> Selector19/1
  Mux19/1 -> Force Estimation/11(Leg Width Right/Left [m m])
  [LLegW] -> Mux19/2
  [RLegW] -> Mux19/1
  [PrimaryLegRoll] -> Force Estimation/9(Primary Leg Roll [rad rad/s])
  [PrimaryLegAngle] -> Force Estimation/8(Primary Leg Angle [rad rad/s])
  [PrimaryLegLength] -> Force Estimation/7(Primary Leg Length [m m/s])
  [q] -> Force Estimation/3(q)
  [TorsoPitch] -> Force Estimation/5(Torso Pitch [rad rad/s])
  [TorsoYaw] -> Force Estimation/6(Torso Yaw [rad rad/s])
  [TorsoRoll] -> Force Estimation/4(Torso Roll [rad rad/s])
  [flight] -> Force Estimation/2(Flight [1/0])
  [RightLeftPrimary] -> Force Estimation/1(Right/Left Primary)
  [ExitingStance] -> Logical Operator/1
  [hopping] -> Logical Operator/2
  [hopping] -> Logical Operator1/2
  [ExitingStance] -> Logical Operator1/1
  Unit Delay2/1 -> [StepCount], Hopping / Steps/2
  [LLegRoll] -> Primary Secondary Leg Swap/19("Left Leg Roll [rad, rad/s]")
  [RLegRoll] -> Primary Secondary Leg Swap/18("Right Leg Roll [rad, rad/s]")
  Primary Secondary Leg Swap/19("Secondary Leg Roll [rad, rad/s]") -> [SecondaryLegRoll]
  Primary Secondary Leg Swap/18("Primary Leg Roll [rad, rad/s]") -> [PrimaryLegRoll]
  Force Estimation/4(GRF XYZ estimates [N N N]) -> GRF XYZ estimates [N N N]/1, [MeasuredGRF]
  Force Estimation/3(Left GRF [X Y Z] [N N N]) -> [LeftLegGRFs]
  [LLateralTorque] -> Gain1/1
  Force Estimation/2(Right GRF [X Y Z] [N N N]) -> [RightLegGRFs]
  Force Estimation/1(Leg Plane Force for Contact Detection [body weight]) -> [ContactDetection]
  Selector28/1 -> [qYaw]
  Selector4/1 -> [qFrontL]
  Selector2/1 -> [qBackL]
  Selector7/1 -> [qFrontR]
  Selector6/1 -> [qBackR]
  Selector1/1 -> [qLatL]
  Selector5/1 -> [qLatR]
  [qBackR] -> Selector16/1
  [dqBackR] -> Selector17/1
  [qFrontR] -> Selector14/1
  [dqFrontR] -> Selector15/1
  Mux2/1 -> R Leg Calculator/1(Front [rad rad/s])
  Mux1/1 -> R Leg Calculator/2(Back [rad rad/s])
  R Leg Calculator/1("Leg Length [m m/s] ") -> [RLegLength]
  R Leg Calculator/2(Leg Angle [rad rad/s]) -> [RLegAngle]
  R Leg Calculator/3(Leg Splay [rad rad/s]) -> [RLegSplay]
  Selector14/1 -> Mux2/1
  Selector15/1 -> Mux2/2
  Selector17/1 -> Mux1/2
  Selector16/1 -> Mux1/1
  q/1 -> Selector6/1, Selector7/1, Selector2/1, Selector4/1, Selector5/1, Selector18/1, Selector28/1, Selector23/1, Selector1/1, [q]
  Selector18/1 -> [qPitch]
  Selector23/1 -> [qRoll]
  [qBackL] -> Selector26/1
  [dqBackL] -> Selector27/1
  [qFrontL] -> Selector24/1
  [dqFrontL] -> Selector25/1
  Mux5/1 -> L Leg Calculator/1(Front [rad rad/s])
  Mux4/1 -> L Leg Calculator/2(Back [rad rad/s])
  L Leg Calculator/1("Leg Length [m m/s] ") -> [LLegLength]
  L Leg Calculator/2(Leg Angle [rad rad/s]) -> [LLegAngle]
  L Leg Calculator/3(Leg Splay [rad rad/s]) -> [LLegSplay]
  Selector24/1 -> Mux5/1
  Selector25/1 -> Mux5/2
  Selector27/1 -> Mux4/2
  Selector26/1 -> Mux4/1
  R Leg Calculator/4(w [m]) -> [RLegW]
  L Leg Calculator/4(w [m]) -> [LLegW]
  Primary Secondary Leg Swap/2(Primary Leg Angle [rad rad/s]) -> [PrimaryLegAngle]
  Primary Secondary Leg Swap/4(Primary Leg w [m]) -> [PrimaryW]
  Primary Secondary Leg Swap/3(Primary Leg Length [m m/s]) -> [PrimaryLegLength]
  [RLegAngle] -> Primary Secondary Leg Swap/2(R Leg Angle [rad rad/s])
  [RLegLength] -> Primary Secondary Leg Swap/3(R Leg Length [m m/s])
  [RLegW] -> Primary Secondary Leg Swap/4(R Leg w [m])
  [LLegAngle] -> Primary Secondary Leg Swap/9(L Leg Angle [rad rad/s])
  [LLegLength] -> Primary Secondary Leg Swap/10(L Leg Length [m m/s])
  [LLegW] -> Primary Secondary Leg Swap/11(L Leg w [m])
  Primary Secondary Leg Swap/10(Secondary Leg Length [rad rad/s]) -> [SecondaryLegLength]
  Primary Secondary Leg Swap/9(Secondary Leg Angle [rad rad/s]) -> [SecondaryLegAngle]
  [qFrontR] -> Demux3/1
  [dqFrontR] -> Demux4/1
  Mux9/1 -> Primary Secondary Leg Swap/5(R Back Joint [rad rad/s])
  Mux10/1 -> Primary Secondary Leg Swap/6(R Back Gear [rad rad/s])
  Mux11/1 -> Primary Secondary Leg Swap/7(R Front Joint [rad rad/s])
  Mux12/1 -> Primary Secondary Leg Swap/8(R Front Gear [rad rad/s])
  Demux3/1 -> Mux11/1
  Demux3/2 -> Mux12/1
  Demux4/1 -> Mux11/2
  Demux4/2 -> Mux12/2
  [dqBackR] -> Demux5/1
  [qBackR] -> Demux6/1
  Demux6/1 -> Mux9/1
  Demux6/2 -> Mux10/1
  Demux5/1 -> Mux9/2
  Demux5/2 -> Mux10/2
  [qFrontL] -> Demux7/1
  [dqFrontL] -> Demux8/1
  Mux16/1 -> Primary Secondary Leg Swap/12(L Back Joint [rad rad/s])
  Mux13/1 -> Primary Secondary Leg Swap/13(L Back Gear [rad rad/s])
  Mux14/1 -> Primary Secondary Leg Swap/14(L Front Joint [rad rad/s])
  Mux15/1 -> Primary Secondary Leg Swap/15(L Front Gear [rad rad/s])
  Demux7/1 -> Mux14/1
  Demux7/2 -> Mux15/1
  Demux8/1 -> Mux14/2
  Demux8/2 -> Mux15/2
  [dqBackL] -> Demux9/1
  [qBackL] -> Demux10/1
  Demux10/1 -> Mux16/1
  Demux10/2 -> Mux13/1
  Demux9/1 -> Mux16/2
  Demux9/2 -> Mux13/2
  [PrimaryBackFrontTorque] -> Primary Secondary Leg Swap/16(Primary Back/Front SEA Torque [Nm Nm])
  [SecondaryBackFrontTorque] -> Primary Secondary Leg Swap/17(Secondary Back/Front SEA Torque [Nm Nm])
  Primary Secondary Leg Swap/5(Primary Back Joint [rad rad/s]) -> [PrimaryBackJoint]
  Primary Secondary Leg Swap/6(Primary Back Gear [rad rad/s]) -> [PrimaryBackGear]
  Primary Secondary Leg Swap/7(Primary Front Joint [rad rad/s]) -> [PrimaryFrontJoint]
  Primary Secondary Leg Swap/8(Primary Front Gear [rad rad/s]) -> [PrimaryFrontGear]
  Primary Secondary Leg Swap/12(Secondary Back Joint [rad rad/s]) -> [SecondaryBackJoint]
  Primary Secondary Leg Swap/13(Secondary Back Gear [rad rad/s]) -> [SecondaryBackGear]
  Primary Secondary Leg Swap/14(Secondary Front Joint [rad rad/s]) -> [SecondaryFrontJoint]
  Primary Secondary Leg Swap/15(Secondary Front Gear [rad rad/s]) -> [SecondaryFrontGear]
  Primary Secondary Leg Swap/11(Secondary Leg w [m]) -> [SecondaryW]
  Primary Secondary Leg Swap/16(R Back/Front SEA Torque [Nm Nm]) -> [RBackFrontTorque]
  Primary Secondary Leg Swap/17(L Back/Front SEA Torque [Nm Nm]) -> [LBackFrontTorque]
  Logical Operator/1 -> Primary Secondary Leg Swap/1(Exiting Stance [1/0])
  Primary Secondary Leg Swap/1(Right/Left Primary [1/0]) -> [RightLeftPrimary]
  Primary and Lateral Behavior/1(Primary Back/Front SEA Torques [Nm] x2) -> [PrimaryBackFrontTorque]
  Primary and Lateral Behavior/3(Primary Force or Position Control [1/0]) -> [PrimaryForcePositionControl]
  [RLateralTorque] -> Gain2/1
  Unit Delay/1 -> Sum1/2
  Sum1/1 -> Unit Delay2/1, Unit Delay/1
  Logical Operator1/1 -> Data Type Conversion/1
  Data Type Conversion/1 -> Sum1/1
  [ExitingStance] -> Exited Stance/Enable
  State Estimation/12(COM Velocity World [m/s m/s m/s]) -> [FootToComVelocityWorld]
  State Estimation/11(COM Position World [m m m]) -> [FootToComPositionWorld]
  [flight] -> State Estimation/15(Flight [1/0])
  [flight] -> Logical Operator4/1
  Logical Operator4/1 -> Logical Operator2/2
  [hopping] -> Logical Operator2/1
  State Estimation/7(Foot to COM Velocity [m/s m/s m/s]) -> [FootToComVelocity]
  State Estimation/6(Foot to COM Position [m m m]) -> [FootToComPosition]
  [TorsoYaw] -> State Estimation/4(Torso Yaw [rad rad/s])
  State Estimation/2("Lateral COM [m, m/s]") -> [Y_dY]
  State Estimation/5(Pelvis to COM Velocity [m/s m/s m/s]) -> [PelvisToComVelocity]
  State Estimation/4(Pelvis to COM Position [m m m]) -> [PelvisToComPosition]
  [LeftLegGRFs] -> State Estimation/13(Left GRF [X Y Z] [N N N])
  [RightLegGRFs] -> State Estimation/12(Right GRF [X Y Z] [N N N])
  Logical Operator2/1 -> State Estimation/11(Enable Kalman Filtering [1/0])
  [RightLeftPrimary] -> State Estimation/1(Right or Left [1/0])
  [RLegAngle] -> State Estimation/8(Right Leg Sagittal Angle [rad rad/s])
  [LLegAngle] -> State Estimation/5(Left Leg Sagittal Angle [rad rad/s])
  [LLegLength] -> State Estimation/7(Left Leg Length [m m/s])
  [LLegRoll] -> State Estimation/6(Left Leg Roll [rad rad/s])
  [RLegRoll] -> State Estimation/9(Right Leg Roll [rad rad/s])
  [TorsoPitch] -> State Estimation/3(Torso Pitch [rad rad/s])
  [TorsoRoll] -> State Estimation/2(Torso Roll [rad rad/s])
  [RLegLength] -> State Estimation/10(Right Leg Length [m m/s])
  State Estimation/3("Vertical COM [m, m/s]") -> [Z_dZ]
  State Estimation/1("Horizontal COM [m, m/s]") -> [X_dX]
  [AccelerationMeasurement] -> State Estimation/14(" Acceleration Measurement [m/s^2] x3")
  State Estimation/8(COM Acceleration [m/s^2] x3) -> [ComAccelerations]
  State Estimation/9(Right Knees to Foot [m m m] x2) -> [RightKneesToFoot], Switch/1
  State Estimation/10(Left Knees to Foot [m m m] x2) -> Switch/3, [LeftKneesToFoot]
  [RightBackAngle] -> State Estimation/16(Right Back [rad rad/s])
  [LeftBackAngle] -> State Estimation/17(Left Back [rad rad/s])
  [RightFrontAngle] -> State Estimation/18(Right Front [rad rad/s])
  [LeftFrontAngle] -> State Estimation/19(Left Front [rad rad/s])
  [RightLeftPrimary] -> Switch/2
  Switch/1 -> [PrimaryKneesToFoot]
  Compute COM Translational Acceleration (IMU uses non-rotating measurement frame)/6(com_acceleration_yawed) -> Demux/1, [AccelerationMeasurement]
  Demux/2 -> COM Acceleration Measurement/2
  Demux/1 -> COM Acceleration Measurement/1
  Demux/3 -> COM Acceleration Measurement/3
  [TorsoPitch] -> Compute COM Translational Acceleration (IMU uses non-rotating measurement frame)/4(torso_pitch)
  [TorsoRoll] -> Compute COM Translational Acceleration (IMU uses non-rotating measurement frame)/3(torso_roll)
  [dqRoll] -> Mux28/1
  [dqPitch] -> Mux28/2
  [dqYaw] -> Mux28/3
  Mux28/1 -> Estimate Angular Accelerations2/1(Angular Velocities [rad/s] x3)
  Enabled [true/false]/1 -> Estimate Angular Accelerations2/2(Enabled), Estimate Angular Accelerations3/2(Enabled)
  Body XYZ Acceleration [m/s^2] x3/1 -> Compute COM Translational Acceleration (IMU uses non-rotating measurement frame)/2(imu_translational_accelerations_body)
  Estimate Angular Accelerations2/1(Angular Accelerations [rad/s^2] x3) -> Compute COM Translational Acceleration (IMU uses non-rotating measurement frame)/1(torso_angular_accelerations)
  [RLegRoll] -> Selector41/1, Compute COM Translational Acceleration (IMU uses non-rotating measurement frame)/9(right_hip_roll)
  [LLegRoll] -> Selector42/1, Compute COM Translational Acceleration (IMU uses non-rotating measurement frame)/10(left_hip_roll)
  Selector41/1 -> Mux30/1
  Selector42/1 -> Mux30/2
  Mux30/1 -> Estimate Angular Accelerations3/1(Angular Velocities [rad/s] x2)
  Estimate Angular Accelerations3/1(Angular Accelerations [rad/s^2] x2) -> Compute COM Translational Acceleration (IMU uses non-rotating measurement frame)/8(hip_roll_accelerations)
  [TorsoYaw] -> Compute COM Translational Acceleration (IMU uses non-rotating measurement frame)/5(torso_yaw)
  Unit Delay5/1 -> Compute COM Translational Acceleration (IMU uses non-rotating measurement frame)/6(com_position_world)
  Unit Delay6/1 -> Compute COM Translational Acceleration (IMU uses non-rotating measurement frame)/7(com_velocity_world)
  Compute World Frame COM Coordinates from Yawed Frame/2(com_velocity_world) -> Unit Delay6/1, Selector44/1
  Compute World Frame COM Coordinates from Yawed Frame/1(com_position_world) -> Unit Delay5/1, Selector43/1
  [X_dX] -> Compute World Frame COM Coordinates from Yawed Frame/1(X_dX)
  [Y_dY] -> Compute World Frame COM Coordinates from Yawed Frame/2(Y_dY)
  [Z_dZ] -> Compute World Frame COM Coordinates from Yawed Frame/3(Z_dZ)
  [TorsoYaw] -> Compute World Frame COM Coordinates from Yawed Frame/4(torso_yaw)
  Mux33/1 -> COM World Frame X/1
  Mux31/1 -> COM World Frame X/2
  [FootToComVelocityWorld] -> Selector45/1
  [FootToComPositionWorld] -> Selector46/1
  Selector43/1 -> Mux33/2
  Selector44/1 -> Mux31/2
  Selector45/1 -> Mux31/1
  Selector46/1 -> Mux33/1
  [SecondaryFrontGear] -> Atrias Swing control/4(Secondary Front Gear [rad rad/s])
  [SecondaryBackGear] -> Atrias Swing control/5(Secondary Back Gear [rad rad/s])
  [RightLeftPrimary] -> Atrias Swing control/6(Right or Left Stance [1 or 0])
  [SecondaryLegRoll] -> Atrias Swing control/7(Secondary Leg Roll [rad rad/s])
  [TorsoRoll] -> Atrias Swing control/11(Torso Roll [rad rad/s])
  [TorsoPitch] -> Atrias Swing control/10(Torso Pitch [rad rad/s])
  [SecondaryLegAngle] -> Atrias Swing control/9(Secondary Leg Angle [rad rad/s])
  [SecondaryLegLength] -> Atrias Swing control/8(Secondary Leg Length [m m/s])
  Mux32/1 -> Atrias Swing control/1(X Desired [m m/s m/s^2])
  Mux25/1 -> Atrias Swing control/2(Y Desired [m m/s m/s^2])
  Mux29/1 -> Atrias Swing control/3(Z Desired [m m/s m/s^2])
  Atrias Swing control/1(Secondary Back/Front Motor Torque [Nm Nm]) -> [SecondaryBackFrontVelocity]
  [Z_dZ] -> Sum2/2
  Constant3/1 -> Sum2/1
  Sum2/1 -> Mux29/1
  [PelvisToComPosition] -> Atrias Swing control/12(Pelvis to COM Position [m m m])
  [PelvisToComVelocity] -> Atrias Swing control/13(Pelvis to COM Velocity [m/s m/s m/s])
  [DesiredSecondaryLegRoll] -> Primary and Lateral Behavior/27(Desired Secondary Leg Roll [rad rad/s])
  Atrias Swing control/2(Desired Swing Beta [rad rad/s]) -> [DesiredSecondaryLegRoll]
  [X_dX] -> Gain/1
  Gain/1 -> Mux32/1
  Constant1/1 -> Switch1/1
  Constant2/1 -> Switch1/3
  [RightLeftPrimary] -> Switch1/2
  Switch1/1 -> Mux25/1
  Constant4/1 -> Mux32/2
  Constant5/1 -> Mux25/2
  Constant6/1 -> Mux29/2
  Force Estimation/6(Primary Axial Leg Force) -> [PrimaryAxialLegForce]
  [PrimaryAxialLegForce] -> Primary and Lateral Behavior/28(Primary Axial Leg Force [N])

== system deadbeat_smm_with_lqr/Control/Compute Body Frame Accelerations ==
  accelerometer [g] x3 : Inport
  Convert to Body Frame IMU Accelerations : MATLAB Function  TreatAsAtomicUnit=on
  IMU Two Pole Filter2 : DiscreteTransferFcn  Numerator=[A_lpf_accelerometer 0 0]  Denominator=[1 B1_lpf_accelerometer B2_lpf_accelerometer]  InitialStates=[0, 0, g; 0, 0, g]*15.277  SampleTime=sample_time
  IMU XYZ Accelerations : Scope
      settings: YMin=-4  YMax=14  SaveName=ScopeData28  SampleInput=on
  Mux : Mux  Inputs=2
  accelerations [m/s^2] x3 : Outport
  wires:
  accelerometer [g] x3/1 -> Convert to Body Frame IMU Accelerations/1(accelerometer)
  Convert to Body Frame IMU Accelerations/1(imu_accelerations) -> Mux/1, IMU Two Pole Filter2/1
  Mux/1 -> IMU XYZ Accelerations/1
  IMU Two Pole Filter2/1 -> Mux/2, accelerations [m/s^2] x3/1

== system deadbeat_smm_with_lqr/Control/Filter Velocities ==
  raw dq : Inport
  Demux : Demux  Outputs=3
  Demux1 : Demux  Outputs=3
  Demux2 : Demux  Outputs=2
  Demux3 : Demux  Outputs=2
  Fourbar : Selector  InputPortWidth=13  Indices=[1 2 3 4 5 6 7 8]
  Fourbar Velocity Filter : Scope  NumInputPorts=4
      settings: YMin=-0.55~-0.4~-0.4~-0.6  YMax=0.25~0.7~0.45~0.5  SaveName=ScopeData14  SampleInput=on
  IMU Two Pole Filter : DiscreteTransferFcn  Numerator=[A_lpf_imu 0 0]  Denominator=[1 B1_lpf_imu B2_lpf_imu]  SampleTime=sample_time
  Lateral : Selector  InputPortWidth=13  Indices=[9 10]
  Lateral Angle Two Pole Filter1 : DiscreteTransferFcn  Numerator=[A_lpf_lateral_angle 0 0]  Denominator=[1 B1_lpf_lateral_angle B2_lpf_lateral_angle]  SampleTime=sample_time
  Lateral Angle Two Pole Filter2 : DiscreteTransferFcn  Numerator=[A_lpf_fourbar_angles 0 0]  Denominator=[1 B1_lpf_fourbar_angles B2_lpf_fourbar_angles]  SampleTime=sample_time
  Leg Roll Velocity Filter : Scope  NumInputPorts=2
      settings: YMin=-0.225~-1.5  YMax=0.175~2.25  SaveName=LegRollFilter  SampleInput=on
  Mux : Mux  Inputs=3
  Mux{25..33} (9 alike) : Mux  Inputs=2
  Selector1 : Selector  InputPortWidth=8  Indices=[1 2]
  Selector2 : Selector  InputPortWidth=8  Indices=[3 4]
  Selector3 : Selector  InputPortWidth=8  Indices=[5 6]
  Selector34 : Selector  InputPortWidth=8  Indices=[1 2]
  Selector35 : Selector  InputPortWidth=8  Indices=[3 4]
  Selector36 : Selector  InputPortWidth=8  Indices=[5 6]
  Selector37 : Selector  InputPortWidth=8  Indices=[7 8]
  Selector4 : Selector  InputPortWidth=8  Indices=[7 8]
  Torso Orientation : Selector  InputPortWidth=13  Indices=[11 12 13]
  Torso Orientation Filter : Scope  NumInputPorts=3
      settings: YMin=-0.2~-0.03~-0.15  YMax=0.125~0.0275~0.15  SaveName=ScopeData13  SampleInput=on
  filtered dq : Outport
  wires:
  Selector1/1 -> Mux30/2
  Selector2/1 -> Mux31/2
  Selector3/1 -> Mux32/2
  Selector4/1 -> Mux33/2
  Demux3/2 -> Mux29/2
  Demux3/1 -> Mux28/2
  Demux2/1 -> Mux28/1
  Demux2/2 -> Mux29/1
  Demux1/3 -> Mux27/2
  Demux1/2 -> Mux26/2
  Demux1/1 -> Mux25/2
  Demux/3 -> Mux27/1
  Demux/2 -> Mux26/1
  Demux/1 -> Mux25/1
  Mux29/1 -> Leg Roll Velocity Filter/2
  Mux28/1 -> Leg Roll Velocity Filter/1
  Selector37/1 -> Mux33/1
  Selector36/1 -> Mux32/1
  Selector35/1 -> Mux31/1
  Fourbar/1 -> Lateral Angle Two Pole Filter2/1, Selector37/1, Selector36/1, Selector35/1, Selector34/1
  Selector34/1 -> Mux30/1
  Mux33/1 -> Fourbar Velocity Filter/4
  Mux31/1 -> Fourbar Velocity Filter/2
  Mux32/1 -> Fourbar Velocity Filter/3
  Mux30/1 -> Fourbar Velocity Filter/1
  Mux26/1 -> Torso Orientation Filter/2
  Mux27/1 -> Torso Orientation Filter/3
  Mux25/1 -> Torso Orientation Filter/1
  Lateral Angle Two Pole Filter1/1 -> Mux/2, Demux3/1
  Torso Orientation/1 -> Demux/1, IMU Two Pole Filter/1
  Lateral/1 -> Lateral Angle Two Pole Filter1/1, Demux2/1
  raw dq/1 -> Lateral/1, Torso Orientation/1, Fourbar/1
  Mux/1 -> filtered dq/1
  IMU Two Pole Filter/1 -> Mux/3, Demux1/1
  Lateral Angle Two Pole Filter2/1 -> Mux/1, Selector1/1, Selector2/1, Selector3/1, Selector4/1

== system deadbeat_smm_with_lqr/Fourbar Gearside Kalman Filter/Pitch Offset ==
  in : Inport
  Constant2 : Constant  Value=torso_centerline_pitch_offset_angle
  Sum : Sum  Inputs=++|
  out : Outport
  wires:
  Constant2/1 -> Sum/1
  Sum/1 -> out/1
  in/1 -> Sum/2

== system deadbeat_smm_with_lqr/Control/Behavior Control/At Least One Stance Detected ==
  Enable : EnablePort  StatesWhenEnabling=reset
  Constant : Constant
  Stance? : Outport  InitialOutput=[0]
  wires:
  Constant/1 -> Stance?/1
